simulink model "ramadan_2022"  (R2021a)
settings: Solver=ode15s  StartTime=0.0  StopTime=10  MaxStep=1e-2  MinStep=1e-20  RelTol=1e-3
StartFcn:
  | tic
StopFcn:
  | toc
  | 
  | 
  | %if GimbalLockFlag
  |  % fprintf(2, 'Almost reached Gimbal Lock of IMU. Simulation stopped.\n')
  | %end
  | 
  | %fprintf('Elapsed time: %4.2f sec (%4.2f%% realtime)\n', a, tout(end)/a*100)
values from neighbouring files (symbols this model uses):
  Balance = pMod(26:29)    [AssignSimulinkParams.m]    (also in assign_parameters.m = param(26:29))
  BalanceTrunkLat = pMod(22:25)    [AssignSimulinkParams.m]    (also in assign_parameters.m = param(22:25))
  BasisStim = pMod(1:11)    [AssignSimulinkParams.m]    (also in assign_parameters.m = param(1:11))
  CompliantLeg = pMod(12:14)    [AssignSimulinkParams.m]    (also in assign_parameters.m = param(12:14))
  CompliantLegLat = pMod(15)    [AssignSimulinkParams.m]    (also in assign_parameters.m = param(15))
  lp1 = 0.45    [nms3D_prep.m]
  lp2 = 0.55    [nms3D_prep.m]
  N = size(x,1)    [cmaes_hg.m]
  PreventKneeOverextension = pMod(16:21)    [AssignSimulinkParams.m]    (also in assign_parameters.m = param(16:21))
  propulsion = pMod(35)    [AssignSimulinkParams.m]    (also in assign_parameters.m = param(35))
  s = x(1:N-1,:).^2 + x(2:N,:).^2    [cmaes_hg.m]
  Target02 = pMod(30)    [AssignSimulinkParams.m]    (also in assign_parameters.m = param(30))
  Target13 = pMod(31:33)    [AssignSimulinkParams.m]    (also in assign_parameters.m = param(31:33))
  theta0 = pMod(34)    [AssignSimulinkParams.m]    (also in assign_parameters.m = param(34))
  WramameiSL_1000 = readmatrix('WSL_1000_Norm_Sigmoid_MSE_cont.csv')    [nms3D_prep.m]
  ZramameiSL_1000 = readmatrix('ZSL_1000_Norm_Sigmoid_MSE_cont.csv')    [nms3D_prep.m]
undefined symbols (not defined in the file or in its folder): ICs, mParams, X, Y, Z
libraries: nesl_utility x110, sm_lib x88, simulink x79, eeGeneralControl x28, robotmaniplib x10, dspinverses x10, robotcorelib x5, dspmathops x3, pid_lib x2, vrlib x1
(part 1 of 9)
settings Model: SimulationMode=rapid-accelerator  Creator=hgeyer  LastModifiedBy=rachidramadan
settings SolverCC: AlgebraicLoopSolver=TrustRegion  DecoupledContinuousIntegration=on  MinimalZcImpactIntegration=on
settings OptimizationCC: EfficientMapNaN2IntZero=off
settings DebuggingCC: ReadBeforeWriteMsg=DisableAll  WriteAfterWriteMsg=DisableAll  WriteAfterReadMsg=DisableAll  IgnoredZcDiagnostic=none  MultiTaskDSMMsg=none  SFMachineParentedDataDiag=warning  ArithmeticOperatorsInVariantConditions=warning
settings HardwareCC: TargetBitPerLong=64  TargetBitPerPointer=64  TargetBitPerSizeT=64  TargetBitPerPtrDiffT=64  TargetLongLongMode=on  TargetIntDivRoundTo=Zero  TargetEndianess=LittleEndian  TargetWordSize=64  TargetHWDeviceType=MATLAB Host  ProdEqTarget=off
settings ModelReferenceCC: UpdateModelReferenceTargets=IfOutOfDate
settings SFSimCC: SFSimEcho=off  SimUseLocalCustomCode=off  CustomCodeUndefinedFunction=UseInterfaceOnly
settings CodeAppCC: MaxIdLength=128
settings ConfigComp: CovScope=ReferencedModels
settings SimscapeCC: SimscapeNormalizeSystem=off
settings ExplorerConfigSet: InternalSimMechanicsExplorerSettings="<ExplorerConfiguration><canonicalview>planar_xy</canonicalview><AnimationSetting><BasePlaybackSpeed>1.0</BasePlaybackSpeed><PlaybackSpeedFactor>1.0</PlaybackSpeedFactor></AnimationSetting><TilePanel><TileInfo><Tiles Columns=\"1\" Count=\"1\" Rows=\"1\"><Column Weight=\"1\"/><Row Weight=\"1\"/><Tile Height=\"1\" Width=\"1\" X=\"0\" Y=\"0\"/></Tiles></TileInfo><SceneInfo><SceneViewer><BGColor><R>0.60000002384185791</R><G>0.60000002384185791</G><B>0.60000002384185791</B></BGColor><Camera><DoPerspective>off</DoPerspective><Position><X>0.597774143722594631</X><Y>0.919449529340500282</Y><Z>14.1815791267909113</Z></Position><Center><X>0.597774143722594631</X><Y>0.919449529340500282</Y><Z>3.38181724401920292e-07</Z></Center><Up><X>0</X><Y>1</Y><Z>0</Z></Up><ViewLimDist>1</ViewLimDist><YLim>1.30566284997374105</YLim><XLim>1.60885047805753101</XLim></Camera></SceneViewer></SceneInfo></TilePanel><MechEditorPanel><Cameras/><GfxPanelCameraMap/><VideoCreator><PlaybackSpeedRatio>1.0</PlaybackSpeedRatio><FrameRate>30</FrameRate><VideoFormat>Motion JPEG AVI</VideoFormat><FrameSize>auto</FrameSize></VideoCreator></MechEditorPanel></ExplorerConfiguration>"

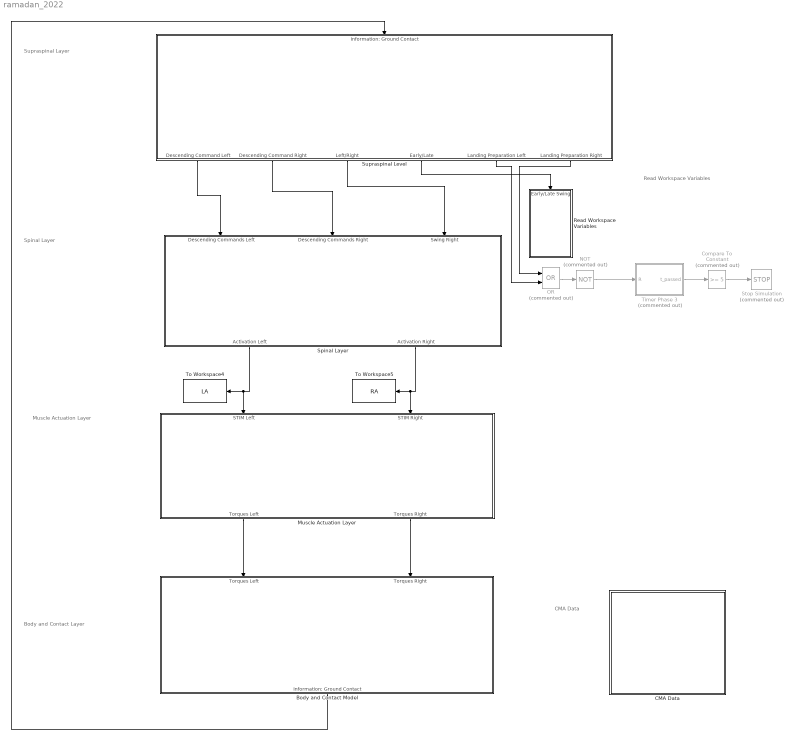
== system ramadan_2022 ==
  note: Spinal Layer
  note: Muscle Actuation Layer
  note: Body and Contact Layer
  note: Supraspinal Layer
  note: CMA Data
  note: Read Workspace Variables
  " Timer Phase 3" : Subsystem  Commented=on
  Body and Contact Model : Subsystem
  CMA Data : Subsystem
  Compare To Constant : simulink/Logic and Bit Operations/Compare To Constant  Commented=on  relop=>=  const=5  OutDataTypeStr=boolean  ZeroCross=off
  Muscle Actuation Layer : Subsystem
  NOT : Logic  Commented=on  Operator=NOT  AllPortsSameDT=off  OutDataTypeStr=boolean
  OR : Logic  Commented=on  Operator=OR  AllPortsSameDT=off  OutDataTypeStr=boolean
  Read Workspace Variables : Subsystem
  Spinal Layer : Subsystem
  Stop Simulation : Stop  Commented=on
  Supraspinal Level : Subsystem
  To Workspace4 : ToWorkspace  VariableName=LA  SampleTime=-1
      settings: Save2DSignal=2-D array (concatenate along first dimension)
  To Workspace5 : ToWorkspace  VariableName=RA  SampleTime=-1
      settings: Save2DSignal=2-D array (concatenate along first dimension)
  wires:
  Spinal Layer/1(Activation Left) -> To Workspace4/1, Muscle Actuation Layer/1(STIM Left)
  Spinal Layer/2(Activation Right) -> To Workspace5/1, Muscle Actuation Layer/2(STIM Right)
  Muscle Actuation Layer/2(Torques Right) -> Body and Contact Model/2(Torques Right)
  Supraspinal Level/1(Descending Command Left) -> Spinal Layer/1(Descending Commands Left)
  Supraspinal Level/2(Descending Command Right) -> Spinal Layer/2(Descending Commands Right)
  Body and Contact Model/1(Information: Ground Contact) -> Supraspinal Level/1(Information: Ground Contact)
  Supraspinal Level/3(Left/Right) -> Spinal Layer/3(Swing Right)
  Supraspinal Level/4(Early/Late) -> Read Workspace Variables/1(Early/Late Swing)
  Muscle Actuation Layer/1(Torques Left) -> Body and Contact Model/1(Torques Left)
  " Timer Phase 3"/1(t_passed) -> Compare To Constant/1
  Compare To Constant/1 -> Stop Simulation/1
  OR/1 -> NOT/1
  Supraspinal Level/6(Landing Preparation Right) -> OR/1
  Supraspinal Level/5(Landing Preparation Left) -> OR/2
  NOT/1 -> " Timer Phase 3"/1(R)

== system ramadan_2022/ Timer Phase 3 ==
  R : Inport
  Clock1 : Clock
  Clock3 : Clock
      settings: Decimation=4
  NOT : Logic  Operator=NOT  AllPortsSameDT=off  OutDataTypeStr=boolean
  Resettable Subsystem : Subsystem  TreatAsAtomicUnit=on
  Sum1 : Sum  Inputs=|+-  InputSameDT=on  SaturateOnIntegerOverflow=on  OutDataTypeStr=Inherit: Same as first input
  Switch2 : Switch  Criteria=u2 > Threshold  RndMeth=Zero
  t_passed : Outport  VectorParamsAs1DForOutWhenUnconnected=off
  wires:
  Clock1/1 -> Sum1/1
  Clock3/1 -> Switch2/3, Resettable Subsystem/1(In1)
  Sum1/1 -> t_passed/1
  R/1 -> NOT/1, Switch2/2
  Switch2/1 -> Sum1/2
  Resettable Subsystem/1(Out1) -> Switch2/1
  NOT/1 -> Resettable Subsystem/Enable

== system ramadan_2022/Body and Contact Model ==
  note: Rigid Body
  note: Contact Model
  note: Vestibular System
  Torques Left : Inport
  Torques Right : Inport  Port=2
  6-DOF Joint IC : sm_lib/Joints/6-DOF Joint  JointMode=Normal  SenseConstraintForce=off  SenseConstraintForceX=off  SenseConstraintForceY=off  SenseConstraintForceZ=off  SenseConstraintTorque=off  SenseConstraintTorqueX=off  SenseConstraintTorqueY=off  SenseConstraintTorqueZ=off  SenseTotalForce=off  SenseTotalForceX=off  SenseTotalForceY=off  SenseTotalForceZ=off  SenseTotalTorque=off  SenseTotalTorqueX=off  SenseTotalTorqueY=off  SenseTotalTorqueZ=off  CompositeWrenchDir=BaseOnFollower  CompositeWrenchFrame=FollowerFrame  PxEquilibriumPosition=0  PxEquilibriumPositionUnits=m  PxSpringStiffness=0  PxSpringStiffnessUnits=N/m  PxDampingCoefficient=0  PxDampingCoefficientUnits=N/(m/s)  PxTorqueActuationMode=NoTorque  PxMotionActuationMode=ComputedMotion  PxSensePosition=off  PxSenseVelocity=off  PxSenseAcceleration=off  PxSenseTorqueForce=off  PxSenseLowerLimitTorqueForce=off  PxSenseUpperLimitTorqueForce=off  PxLowerLimitSpecify=off  PxLowerLimitBound=-1  PxLowerLimitBoundUnits=m  PxLowerLimitStiffness=1e6  PxLowerLimitStiffnessUnits=N/m  PxLowerLimitDamping=1e3  PxLowerLimitDampingUnits=N/(m/s)  PxLowerLimitTransitionRegionWidth=1e-4  PxLowerLimitTransitionRegionWidthUnits=m  PxUpperLimitSpecify=off  PxUpperLimitBound=1  PxUpperLimitBoundUnits=m  PxUpperLimitStiffness=1e6  PxUpperLimitStiffnessUnits=N/m  PxUpperLimitDamping=1e3  PxUpperLimitDampingUnits=N/(m/s)  PxUpperLimitTransitionRegionWidth=1e-4  PxUpperLimitTransitionRegionWidthUnits=m  PxPositionTargetSpecify=on  PxPositionTargetPriority=High  PxPositionTargetValue=ICs.trunk.x0  PxPositionTargetValueUnits=m  PxVelocityTargetSpecify=on  PxVelocityTargetPriority=High  PxVelocityTargetValue=ICs.trunk.vx0  PxVelocityTargetValueUnits=m/s  PyEquilibriumPosition=0  PyEquilibriumPositionUnits=m  PySpringStiffness=0  PySpringStiffnessUnits=N/m  PyDampingCoefficient=0  PyDampingCoefficientUnits=N/(m/s)  PyTorqueActuationMode=NoTorque  PyMotionActuationMode=ComputedMotion  PySensePosition=off  PySenseVelocity=off  PySenseAcceleration=off  PySenseTorqueForce=off  PySenseLowerLimitTorqueForce=off  PySenseUpperLimitTorqueForce=off  PyLowerLimitSpecify=off  PyLowerLimitBound=-1  PyLowerLimitBoundUnits=m  PyLowerLimitStiffness=1e6  PyLowerLimitStiffnessUnits=N/m  PyLowerLimitDamping=1e3  PyLowerLimitDampingUnits=N/(m/s)  PyLowerLimitTransitionRegionWidth=1e-4  PyLowerLimitTransitionRegionWidthUnits=m  PyUpperLimitSpecify=off  PyUpperLimitBound=1  PyUpperLimitBoundUnits=m  PyUpperLimitStiffness=1e6  PyUpperLimitStiffnessUnits=N/m  PyUpperLimitDamping=1e3  PyUpperLimitDampingUnits=N/(m/s)  PyUpperLimitTransitionRegionWidth=1e-4  PyUpperLimitTransitionRegionWidthUnits=m  PyPositionTargetSpecify=on  PyPositionTargetPriority=High  PyPositionTargetValue=ICs.trunk.y0  PyPositionTargetValueUnits=m  PyVelocityTargetSpecify=off  PyVelocityTargetPriority=High  PyVelocityTargetValue=0  PyVelocityTargetValueUnits=m/s  PzEquilibriumPosition=0  PzEquilibriumPositionUnits=m  PzSpringStiffness=0  PzSpringStiffnessUnits=N/m  PzDampingCoefficient=0  PzDampingCoefficientUnits=N/(m/s)  PzTorqueActuationMode=NoTorque  PzMotionActuationMode=ComputedMotion  PzSensePosition=off  PzSenseVelocity=off  PzSenseAcceleration=off  PzSenseTorqueForce=off  PzSenseLowerLimitTorqueForce=off  PzSenseUpperLimitTorqueForce=off  PzLowerLimitSpecify=off  PzLowerLimitBound=-1  PzLowerLimitBoundUnits=m  PzLowerLimitStiffness=1e6  PzLowerLimitStiffnessUnits=N/m  PzLowerLimitDamping=1e3  PzLowerLimitDampingUnits=N/(m/s)  PzLowerLimitTransitionRegionWidth=1e-4  PzLowerLimitTransitionRegionWidthUnits=m  PzUpperLimitSpecify=off  PzUpperLimitBound=1  PzUpperLimitBoundUnits=m  PzUpperLimitStiffness=1e6  PzUpperLimitStiffnessUnits=N/m  PzUpperLimitDamping=1e3  PzUpperLimitDampingUnits=N/(m/s)  PzUpperLimitTransitionRegionWidth=1e-4  PzUpperLimitTransitionRegionWidthUnits=m  PzPositionTargetSpecify=on  PzPositionTargetPriority=High  PzPositionTargetValue=ICs.trunk.z0  PzPositionTargetValueUnits=m  PzVelocityTargetSpecify=on  PzVelocityTargetPriority=High  PzVelocityTargetValue=ICs.trunk.vz0  PzVelocityTargetValueUnits=m/s  SphDefPosRotationMethod=None  SphDefPosRotationAngleUnits=deg  SphDefPosRotationStandardAxis=+Z  SphDefPosRotationAngle=0.0  SphDefPosRotationArbitraryAxis=[0 0 1]  SphDefPosFollAlignAxisA=+X  SphDefPosBaseAlignAxisA=+Y  SphDefPosFollAlignAxisB=+Y  SphDefPosBaseAlignAxisB=+Z  SphDefPosRotationSequenceAxes=FollowerAxes  SphDefPosRotationSequence=XYX  SphDefPosRotationSequenceAngles=[0 0 0]  SphDefPosRotationSequenceAnglesUnits=deg  SphDefPosRotationMatrix=[1 0 0; 0 1 0; 0 0 1]  SphEqPosRotationMethod=None  SphEqPosRotationAngleUnits=deg  SphEqPosRotationStandardAxis=+Y  SphEqPosRotationAngle=0.0  SphEqPosRotationArbitraryAxis=[0 0 1]  SphEqPosFollAlignAxisA=+X  SphEqPosBaseAlignAxisA=+Y  SphEqPosFollAlignAxisB=+Y  SphEqPosBaseAlignAxisB=+Z  SphEqPosRotationSequenceAxes=FollowerAxes  SphEqPosRotationSequence=XYZ  SphEqPosRotationSequenceAngles=[0 0 -0.3]  SphEqPosRotationSequenceAnglesUnits=rad  SphEqPosRotationMatrix=[1 0 0; 0 1 0; 0 0 1]  SphSpringStiffness=0  SphSpringStiffnessUnits=N*m/deg  SphDampingCoefficient=0  SphDampingCoefficientUnits=N*m/(deg/s)  SphActuateTorqueX=off  SphActuateTorqueY=off  SphActuateTorqueZ=off  SphActuateTorque=on  SphTorqueActuationMode=NoTorque  SphMotionActuationMode=ComputedMotion  SphActuationFrame=BaseFrame  SphSensePosition=off  SphSenseVelocityX=off  SphSenseVelocityY=off  SphSenseVelocityZ=off  SphSenseVelocity=off  SphSenseAccelerationX=off  SphSenseAccelerationY=off  SphSenseAccelerationZ=off  SphSenseAcceleration=off  SphSenseTorqueX=off  SphSenseTorqueY=off  SphSenseTorqueZ=off  SphSenseTorqueForce=off  SphSenseLowerLimitTorqueMag=off  SphSenseUpperLimitTorqueMag=off  SphSensingFrame=BaseFrame  SphLowerLimitSpecify=off  SphLowerLimitBound=15  SphLowerLimitBoundUnits=deg  SphLowerLimitStiffness=1e4  SphLowerLimitStiffnessUnits=N*m/deg  SphLowerLimitDamping=10  SphLowerLimitDampingUnits=N*m/(deg/s)  SphLowerLimitTransitionRegionWidth=0.1  SphLowerLimitTransitionRegionWidthUnits=deg  SphUpperLimitSpecify=off  SphUpperLimitBound=45  SphUpperLimitBoundUnits=deg  SphUpperLimitStiffness=1e4  SphUpperLimitStiffnessUnits=N*m/deg  SphUpperLimitDamping=10  SphUpperLimitDampingUnits=N*m/(deg/s)  SphUpperLimitTransitionRegionWidth=0.1  SphUpperLimitTransitionRegionWidthUnits=deg  SphPositionTargetRotationMethod=RotationSequence  SphPositionTargetRotationAngleUnits=deg  SphPositionTargetRotationStandardAxis=+Z  SphPositionTargetRotationAngle=0.0  SphPositionTargetRotationArbitraryAxis=[0 0 1]  SphPositionTargetFollAlignAxisA=+X  SphPositionTargetBaseAlignAxisA=+Y  SphPositionTargetFollAlignAxisB=+Y  SphPositionTargetBaseAlignAxisB=+Z  SphPositionTargetRotationSequenceAxes=BaseAxes  SphPositionTargetRotationSequence=XZY  SphPositionTargetRotationSequenceAngles=[ICs.trunk.qR0 ICs.trunk.qP0 ICs.trunk.qY0 ]  SphPositionTargetRotationSequenceAnglesUnits=rad  SphPositionTargetRotationMatrix=[1 0 0; 0 1 0; 0 0 1]  SphPositionTargetSpecify=on  SphPositionTargetPriority=High  SphVelocityTargetValue=[ICs.trunk.qR0 ICs.trunk.qP0 ICs.trunk.qY0 ]  SphVelocityTargetValueUnits=deg/s  SphVelocityTargetSpecify=on  SphVelocityTargetPriority=High  SphVelocityTargetInFollowerFrame=on
  Clock : Clock
  Compare To Constant : simulink/Logic and Bit Operations/Compare To Constant  relop=<=  const=0.05  OutDataTypeStr=boolean
  Constant : Constant  Value=0
  External Force and Torque : sm_lib/Forces and Torques/External Force and Torque  ForceResolutionFrame=AttachedFrame  EnableForceX=on  EnableForceY=off  EnableForceZ=off  EnableForce=off  TorqueResolutionFrame=AttachedFrame  EnableTorqueX=off  EnableTorqueY=off  EnableTorqueZ=off  EnableTorque=off
  L Leg : Subsystem
  Minus : Sum  Inputs=-+
  PID Controller : pid_lib/PID Controller  Controller=P  Form=Parallel  TimeDomain=Continuous-time  UseExternalTs=off  SampleTime=-1  IntegratorMethod=Forward Euler  FilterMethod=Forward Euler  ControllerParametersSource=internal  P=7000  I=1  D=0  UseFilter=on  N=100  TunerSelectOption=Transfer Function Based (PID Tuner App)  ZeroCross=off  InitialConditionSource=internal  InitialConditionForIntegrator=0  InitialConditionForFilter=0  DifferentiatorICPrevScaledInput=0  ExternalReset=none  TrackingMode=off  Kt=1  LimitOutput=off  SatLimitsSource=internal  UpperSaturationLimit=inf  LowerSaturationLimit=-inf  LinearizeAsGain=on  AntiWindupMode=none  Kb=1  POutMin=[]  POutMax=[]  IOutMin=[]  IOutMax=[]  DOutMin=[]  DOutMax=[]  NOutMin=[]  NOutMax=[]  SumOutMin=[]  SumOutMax=[]  SaturationOutMin=[]  SaturationOutMax=[]  PParamMin=[]  PParamMax=[]  IParamMin=[]  IParamMax=[]  DParamMin=[]  DParamMax=[]  NParamMin=[]  NParamMax=[]  KbParamMin=[]  KbParamMax=[]  KtParamMin=[]  KtParamMax=[]  KbOutMin=[]  KbOutMax=[]  KtOutMin=[]  KtOutMax=[]  IntegratorOutMin=[]  IntegratorOutMax=[]  FilterOutMin=[]  FilterOutMax=[]  SumI1OutMin=[]  SumI1OutMax=[]  SumI2OutMin=[]  SumI2OutMax=[]  SumI3OutMin=[]  SumI3OutMax=[]  SumI4OutMin=[]  SumI4OutMax=[]  SumDOutMin=[]  SumDOutMax=[]  DifferentiatorOutMin=[]  DifferentiatorOutMax=[]  FilterDiffOutCoefMin=[]  FilterDiffOutCoefMax=[]  ReciprocalOutMin=[]  ReciprocalOutMax=[]  SumDenOutMin=[]  SumDenOutMax=[]  SumNumOutMin=[]  SumNumOutMax=[]  DivideOutMin=[]  DivideOutMax=[]  UdiffTsProdOutMin=[]  UdiffTsProdOutMax=[]  NTsProdOutMin=[]  NTsProdOutMax=[]  UintegralTsProdOutMin=[]  UintegralTsProdOutMax=[]  UngainTsProdOutMin=[]  UngainTsProdOutMax=[]  IntegratorContinuousStateAttributes=''  IntegratorStateMustResolveToSignalObject=off  IntegratorRTWStateStorageClass=Auto  FilterContinuousStateAttributes=''  FilterStateMustResolveToSignalObject=off  FilterRTWStateStorageClass=Auto  ParallelPVariant=InternalParameters  IdealPVariant=Disabled  IVariant=Disabled  DVariant=Disabled  IntegratorVariant=Disabled  SatVariant=Disabled  AWVariant=Disabled  PCopyVariant=Disabled  TRVariant=Disabled  FdbkBlocksVariant=Forward  IdealPFdbkVariant=Disabled  SatFdbkVariant=Disabled  DerivativeFilterVariant=Disabled  NVariant=Disabled  NCopyVariant=Disabled_SignalSpec  FilterICVariant=Disabled  IntegratorICVariant=Disabled  ExternalResetVariant=Disabled  TRSumVariant=Passthrough  SumFdbkVariant=Disabled  SumVariant=Passthrough_P  TsampFilterVariant=InternalTs  TsampNgainVariant=Passthrough  TsampIntegralVariant=Disabled_SignalSpec  ExternalSaturationOutDataTypeStr=Inherit: Same as second input
  R Leg : Subsystem
  Selector : Selector  InputPortWidth=3  IndexOptions=Index vector (dialog)  Indices=[1]  OutputSizes=1
  Sensor Left Ankle : Subsystem
  Sensor Left Ankle1 : Subsystem
  Simulink-PS Converter : nesl_utility/Simulink-PS Converter  PhysicalDomain=network_engine_domain  SubClassName=ps_input  LeftPortType=input  RightPortType=output  PseudoPeriodic=off  Frequencies=[]  NoiseDistribution=none  NoiseParameters=[]  Unit=1  AffineConversion=off  FilteringAndDerivatives=provide  SimscapeFilterOrder=1  InputFilterTimeConstant=0.001  UdotUserProvided=0
      settings: SourceProductBaseCode=PW,SS
  Subsystem : Subsystem
  Switch : Switch  Criteria=u2 > Threshold
  Terminator : Terminator
  Terminator1 : Terminator
  To Workspace1 : ToWorkspace  VariableName=Rlegq  SampleTime=-1
      settings: Save2DSignal=2-D array (concatenate along first dimension)
  To Workspace2 : ToWorkspace  VariableName=Llegdq  SampleTime=-1
      settings: Save2DSignal=2-D array (concatenate along first dimension)
  To Workspace3 : ToWorkspace  VariableName=Llegq  SampleTime=-1
      settings: Save2DSignal=2-D array (concatenate along first dimension)
  Trunk (floating base) : Subsystem
  Vestibular System : Subsystem
  World Frame : Subsystem
  Information: Ground Contact : Outport
  tag scope: LHL=global, LHR=global, Llegddq=global, Llegdq=global, Llegq=global, Rlegddq=global, Rlegdq=global, Rlegq=global
  wires:
  R Leg/4("Joint Velocities Right [rad/s] ") -> [Rlegdq]
  R Leg/5(Joint Accelerations Right [rad/s^2]) -> [Rlegddq]
  R Leg/3(Joint Angles Right [rad]) -> To Workspace1/1, [Rlegq]
  L Leg/3(Joint Angles Left [rad]) -> To Workspace3/1, [Llegq]
  L Leg/5(Joint Accelerations Left [rad/s^2]) -> [Llegddq]
  L Leg/4("Joint Velocities Left [rad/s] ") -> To Workspace2/1, [Llegdq]
  R Leg/2(Position Right Ankle [m]) -> Vestibular System/1(Ankle Position Right [m])
  L Leg/2(" Position Left Ankle [m]") -> Vestibular System/2(Ankle Position Left [m])
  Subsystem/1(Information: Ground Contact) -> Information: Ground Contact/1
  L Leg/1(Rotation Matrix Left Knee (world)) -> Terminator/1
  R Leg/1(Rotation Matrix Right Knee (World)) -> Terminator1/1
  Torques Right/1 -> R Leg/1(Torques [Nm])
  Torques Left/1 -> L Leg/1(Torques [Nm])
  Sensor Left Ankle/1(Position [m]) -> [LHL]
  Sensor Left Ankle1/1(Position [m]) -> [LHR]
  [CoM_Velocity] -> Selector/1
  Selector/1 -> Minus/1
  [v_init] -> Minus/2
  Minus/1 -> PID Controller/1
  PID Controller/1 -> Switch/1
  Constant/1 -> Switch/3
  Clock/1 -> Compare To Constant/1
  Compare To Constant/1 -> Switch/2
  Switch/1 -> Simulink-PS Converter/1
  connections:
  Trunk (floating base)/RConn1 -- Vestibular System/LConn3 -- L Leg/LConn1
  World Frame/RConn1 -- Subsystem/LConn1 -- 6-DOF Joint IC/LConn1
  L Leg/RConn1 -- Subsystem/RConn1
  L Leg/RConn2 -- Sensor Left Ankle/LConn1 -- Subsystem/RConn2
  L Leg/RConn3 -- Subsystem/RConn3
  L Leg/RConn4 -- Subsystem/RConn4
  R Leg/RConn3 -- Subsystem/RConn7
  R Leg/RConn4 -- Subsystem/RConn8
  Vestibular System/LConn2 -- R Leg/LConn1 -- Trunk (floating base)/RConn2
  6-DOF Joint IC/RConn1 -- Vestibular System/LConn1 -- Trunk (floating base)/LConn1 -- External Force and Torque/RConn1
  Subsystem/RConn6 -- Sensor Left Ankle1/LConn1 -- R Leg/RConn1
  R Leg/RConn2 -- Subsystem/RConn5
  External Force and Torque/LConn1 -- Simulink-PS Converter/RConn1

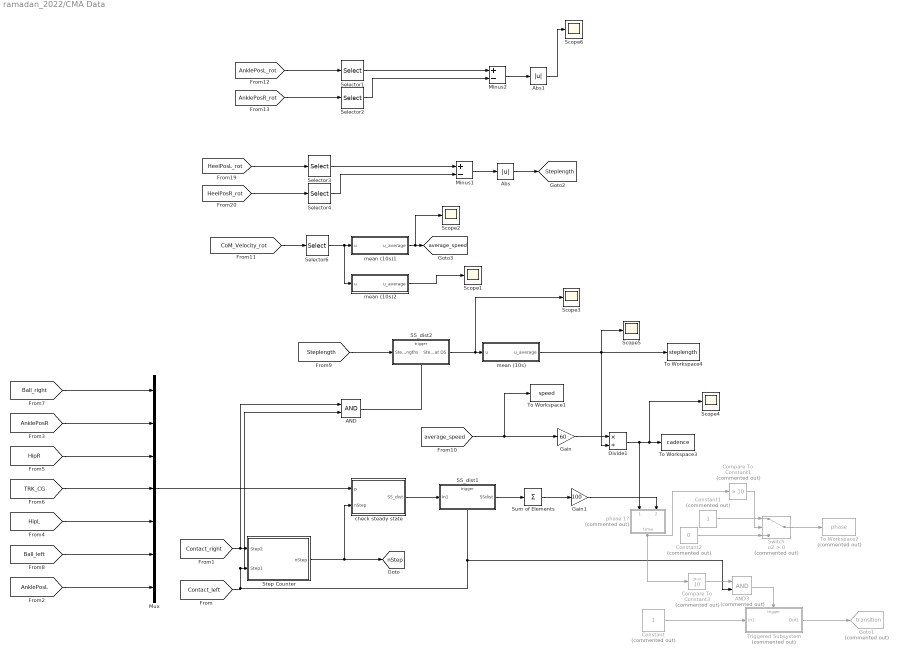
== system ramadan_2022/CMA Data ==
  AND : Logic  AllPortsSameDT=off  OutDataTypeStr=boolean
  AND3 : Logic  Commented=on  AllPortsSameDT=off  OutDataTypeStr=boolean
  Abs : Abs  ZeroCross=off
  Abs1 : Abs  ZeroCross=off
  Compare To Constant1 : simulink/Logic and Bit Operations/Compare To Constant  Commented=on  relop=>  const=10  OutDataTypeStr=boolean
  Compare To Constant3 : simulink/Logic and Bit Operations/Compare To Constant  Commented=on  relop=>=  const=10  OutDataTypeStr=boolean
  Constant : Constant  Commented=on  VectorParams1D=off  SampleTime=-1
  Constant1 : Constant  Commented=on
  Constant2 : Constant  Commented=on  Value=0
  Divide1 : Product  Inputs=*/
  Gain : Gain  Gain=60
  Gain1 : Gain  Gain=100
  Goto1 : Goto  Commented=on  GotoTag=transition  TagVisibility=global
  Minus1 : Sum  Inputs=+-
  Minus2 : Sum  Inputs=+-
  Mux : Mux  Inputs=7
  SS_dist1 : Subsystem  TreatAsAtomicUnit=on
  SS_dist2 : Subsystem  TreatAsAtomicUnit=on
  Scope{1..6} (6 alike) : Scope
  Selector{1..4,6} (5 alike) : Selector  InputPortWidth=3  IndexOptions=Index vector (dialog)  Indices=[1]  OutputSizes=1
  Step Counter : Subsystem
  Sum of Elements : Sum  Inputs=+
  Switch : Switch  Commented=on  Criteria=u2 > Threshold
  To Workspace1 : ToWorkspace  VariableName=speed  SampleTime=-1
      settings: Save2DSignal=2-D array (concatenate along first dimension)
  To Workspace2 : ToWorkspace  Commented=on  VariableName=phase  SampleTime=-1
      settings: Save2DSignal=2-D array (concatenate along first dimension)
  To Workspace3 : ToWorkspace  VariableName=cadence  SampleTime=-1
      settings: Save2DSignal=2-D array (concatenate along first dimension)
  To Workspace4 : ToWorkspace  VariableName=steplength  SampleTime=-1
      settings: Save2DSignal=2-D array (concatenate along first dimension)
  Triggered Subsystem : Subsystem  Commented=on  TreatAsAtomicUnit=on
  check steady state : Subsystem
  mean (10s) : Subsystem
  mean (10s)1 : Subsystem
  mean (10s)2 : Subsystem
  phase 1? : Subsystem  Commented=on
  tag scope: Steplength=global, average_speed=global, nStep=global
  wires:
  Step Counter/1(nStep) -> check steady state/2(nStep), [nStep]
  [Contact_left] -> AND/2, Step Counter/2(Step1), SS_dist1/Trigger, AND3/2
  [Contact_right] -> AND/1, Step Counter/1(Step2)
  [Ball_right] -> Mux/1
  [AnklePosR] -> Mux/2
  [HipR] -> Mux/3
  [TRK_CG] -> Mux/4
  [HipL] -> Mux/5
  [Ball_left] -> Mux/6
  [AnklePosL] -> Mux/7
  Mux/1 -> check steady state/1(p)
  check steady state/1(SS_dist) -> SS_dist1/1(In1)
  [Steplength] -> SS_dist2/1(Steplengths)
  SS_dist2/1(Steplength at DS) -> Scope3/1, mean (10s)/1(u)
  AND/1 -> SS_dist2/Trigger
  mean (10s)/1(u_average) -> Divide1/2, To Workspace4/1, Scope5/1
  [average_speed] -> To Workspace1/1, Gain/1
  Divide1/1 -> Scope4/1, To Workspace3/1, phase 1?/1(cadence)
  Gain/1 -> Divide1/1
  SS_dist1/1(SSdist) -> Sum of Elements/1
  Sum of Elements/1 -> Gain1/1
  Compare To Constant3/1 -> AND3/1
  AND3/1 -> Triggered Subsystem/Trigger
  Triggered Subsystem/1(Out1) -> Goto1/1
  Constant/1 -> Triggered Subsystem/1(In1)
  Gain1/1 -> phase 1?/2(stability)
  phase 1?/1(time) -> Compare To Constant1/1, Compare To Constant3/1
  Constant1/1 -> Switch/1
  Constant2/1 -> Switch/3
  Switch/1 -> To Workspace2/1
  Compare To Constant1/1 -> Switch/2
  Selector3/1 -> Minus1/1
  [HeelPosL_rot] -> Selector3/1
  Selector4/1 -> Minus1/2
  [HeelPosR_rot] -> Selector4/1
  Minus1/1 -> Abs/1
  Abs/1 -> [Steplength]
  [CoM_Velocity_rot] -> Selector6/1
  mean (10s)1/1(u_average) -> Scope2/1, [average_speed]
  Selector6/1 -> mean (10s)2/1(u), mean (10s)1/1(u)
  Selector2/1 -> Minus2/2
  Abs1/1 -> Scope6/1
  [AnklePosL_rot] -> Selector1/1
  [AnklePosR_rot] -> Selector2/1
  Selector1/1 -> Minus2/1
  Minus2/1 -> Abs1/1
  mean (10s)2/1(u_average) -> Scope1/1

== system ramadan_2022/Muscle Actuation Layer ==
  note: Muscle Actuation Layer
  STIM Left : Inport
  STIM Right : Inport  Port=2
  Muscles Left : Subsystem
  Muscles Right : Subsystem
  Mux : Mux
  Mux1 : Mux
  Torques Left : Outport
  Torques Right : Outport  Port=2
  tag scope: BalanceTorqueLeft=global, stance_torque_left_norm=global, stance_torque_right_norm=global
  wires:
  STIM Left/1 -> Muscles Left/1(STIM Left)
  STIM Right/1 -> Muscles Right/1(STIM Right)
  Muscles Left/1(tauHipPitchL) -> Mux/1
  Muscles Left/2(tauHipRollL) -> Mux/2
  Muscles Right/1(tauHipPitchR) -> Mux1/1
  Muscles Right/2(tauHipRollR) -> Mux1/2
  Muscles Left/4(tauHipAnkleL) -> Mux/4
  Muscles Right/3(tauKneeR) -> Mux1/3
  Muscles Left/3(tauKneeL) -> Mux/3
  Muscles Right/4(tauHipAnkleR) -> Mux1/4
  Mux/1 -> Torques Left/1
  Mux1/1 -> Torques Right/1
  Muscles Right/5(Leg Torque) -> [stance_torque_right_norm]
  Muscles Left/5("Leg Torque ") -> [stance_torque_left_norm]

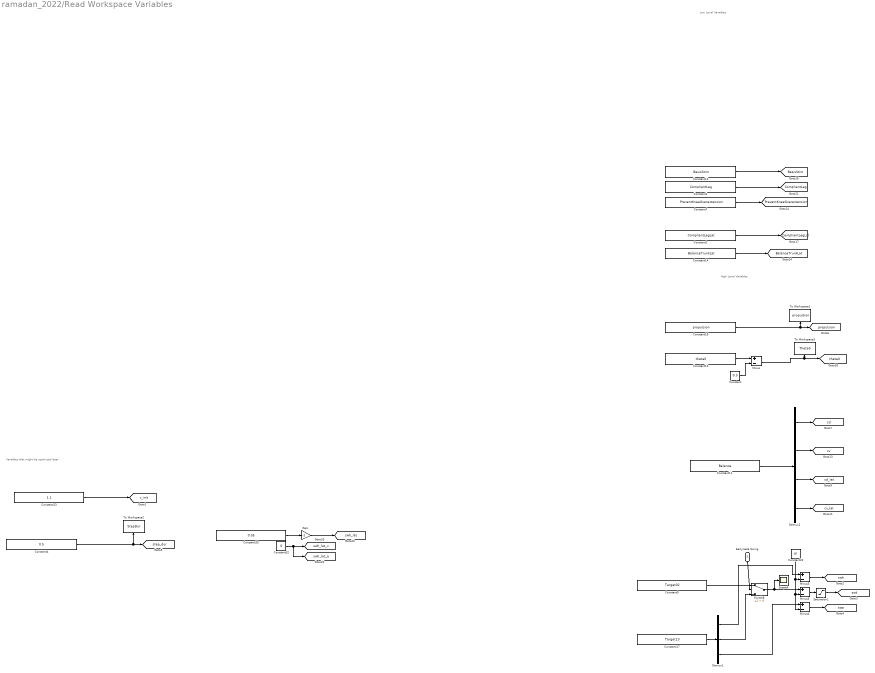
== system ramadan_2022/Read Workspace Variables ==
  note: Low Level Variables
  note: High Level Variables
  note: Variables that might be optimized later
  Early/Late Swing : Inport
  Constant : Constant  Value=0.3
  Constant1 : Constant  Value=CompliantLeg
  Constant10 : Constant  Value=theta0
  Constant11 : Constant  Value=Balance
  Constant12 : Constant  Value=BasisStim
  Constant14 : Constant  Value=BalanceTrunkLat
  Constant16 : Constant  Value=propulsion
  Constant17 : Constant  Value=Target13
  Constant2 : Constant  Value=CompliantLegLat
  Constant22 : Constant  Value=pi
  Constant23 : Constant  Value=1.1
  Constant32 : Constant  Value=0
  Constant33 : Constant  Value=0.05
  Constant4 : Constant  Value=0.5
  Constant7 : Constant  Value=PreventKneeOverextension
  Constant9 : Constant  Value=Target02
  Demux1 : Demux  Outputs=3
  Demux2 : Demux
  Gain : Gain  Gain=-1
  Minus{,3..5} (4 alike) : Sum  Inputs=+-
  Saturation1 : Saturate  UpperLimit=pi  LowerLimit=0  ZeroCross=off
  Scope4 : Scope
  Switch8 : Switch  Criteria=u2 > Threshold
  To Workspace1 : ToWorkspace  VariableName=propulsion  SampleTime=-1
      settings: Save2DSignal=2-D array (concatenate along first dimension)
  To Workspace2 : ToWorkspace  VariableName=StepDur  SampleTime=-1
      settings: Save2DSignal=2-D array (concatenate along first dimension)
  To Workspace3 : ToWorkspace  VariableName=Theta0  SampleTime=-1
      settings: Save2DSignal=2-D array (concatenate along first dimension)
  tag scope: BalanceTrunkLat=global, BasisStim=global, CompliantLeg=global, CompliantLegLat=global, PreventKneeOverextension=global, cd=global, cd_lat=global, cv=global, cv_lat=global, propulsion=global, step_dur=global, swa=global, swh=global, swh_lat=global, swh_lat_a=global, swh_lat_v=global, swk=global, theta0=global, v_init=global
  wires:
  Constant1/1 -> [CompliantLeg]
  Constant12/1 -> [BasisStim]
  Constant7/1 -> [PreventKneeOverextension]
  Demux2/3 -> [cd_lat]
  Demux2/2 -> [cv]
  Demux2/4 -> [cv_lat]
  Demux2/1 -> [cd]
  Constant2/1 -> [CompliantLegLat]
  Constant14/1 -> [BalanceTrunkLat]
  Constant33/1 -> Gain/1
  Constant16/1 -> [propulsion], To Workspace1/1
  Constant4/1 -> To Workspace2/1, [step_dur]
  Constant32/1 -> [swh_lat_a], [swh_lat_v]
  Gain/1 -> [swh_lat]
  Constant23/1 -> [v_init]
  Constant17/1 -> Demux1/1
  Constant9/1 -> Switch8/1
  Demux1/1 -> Minus3/1
  Demux1/2 -> Switch8/3
  Switch8/1 -> Minus5/1, Scope4/1
  Demux1/3 -> Minus4/1
  Minus3/1 -> [swh]
  Minus4/1 -> [swa]
  Constant22/1 -> Minus4/2, Minus5/2, Minus3/2
  Early/Late Swing/1 -> Switch8/2
  Constant11/1 -> Demux2/1
  Minus5/1 -> Saturation1/1
  Saturation1/1 -> [swk]
  Constant10/1 -> Minus/1
  Constant/1 -> Minus/2
  Minus/1 -> To Workspace3/1, [theta0]

== system ramadan_2022/Spinal Layer ==
  Descending Commands Left : Inport
  Descending Commands Right : Inport  Port=2
  Swing Right : Inport  Port=3
  Add1 : Sum
  Add2 : Sum
  Saturation1 : Saturate  UpperLimit=1  LowerLimit=0.001  ZeroCross=off
  Saturation2 : Saturate  UpperLimit=1  LowerLimit=0.001  ZeroCross=off
  Stance Leg Control Left : Subsystem
  Stance Leg Control Right : Subsystem
  Stretch Reflex for Swing Leg Control : Subsystem
  Switch : Switch  Criteria=u2 > Threshold
  Switch1 : Switch  Criteria=u2 > Threshold
  Activation Left : Outport
  Activation Right : Outport  Port=2
  wires:
  Descending Commands Right/1 -> Stretch Reflex for Swing Leg Control/2(Descending Commands Right)
  Descending Commands Left/1 -> Stretch Reflex for Swing Leg Control/1(Descending Commands Left)
  Stance Leg Control Left/1(Activation Left) -> Add1/2
  Stance Leg Control Right/1(Activation Right) -> Add2/2
  Switch1/1 -> Saturation1/1
  Switch/1 -> Saturation2/1
  Add1/1 -> Switch1/1
  Add2/1 -> Switch/3
  Saturation1/1 -> Activation Left/1
  Saturation2/1 -> Activation Right/1
  Stretch Reflex for Swing Leg Control/2(Activation Right) -> Add2/1, Switch/1
  Stretch Reflex for Swing Leg Control/1(Activation Left) -> Add1/1, Switch1/3
  Swing Right/1 -> Switch/2, Switch1/2, Stance Leg Control Right/1(Left/Right), Stance Leg Control Left/1(Left/Right)

== system ramadan_2022/Supraspinal Level ==
  note: Finite State Machine
  note: Computing Descending Commands for Swing Leg Control
  Information: Ground Contact : Inport
  Early/ Late : Logic  Operator=OR  AllPortsSameDT=off  OutDataTypeStr=boolean
  Finite State Machine : Subsystem
  Landing Preperation : Logic  Operator=OR  AllPortsSameDT=off  OutDataTypeStr=boolean
  Left/ Right : Logic  Operator=OR  Inputs=3  AllPortsSameDT=off  OutDataTypeStr=boolean
  Subsystem : Subsystem
  Terminator : Terminator
  To Workspace1 : ToWorkspace  VariableName=LateRight  SampleTime=-1
      settings: Save2DSignal=2-D array (concatenate along first dimension)
  To Workspace2 : ToWorkspace  VariableName=EarlyRight  SampleTime=-1
      settings: Save2DSignal=2-D array (concatenate along first dimension)
  To Workspace3 : ToWorkspace  VariableName=EarlyLeft  SampleTime=-1
      settings: Save2DSignal=2-D array (concatenate along first dimension)
  To Workspace4 : ToWorkspace  VariableName=Contact  SampleTime=-1
      settings: Save2DSignal=2-D array (concatenate along first dimension)
  Descending Command Left : Outport
  Descending Command Right : Outport  Port=2
  Left/Right : Outport  Port=3
  Early/Late : Outport  Port=4
  Landing Preparation Left : Outport  Port=5
  Landing Preparation Right : Outport  Port=6
  wires:
  Finite State Machine/3(Early Left Swing) -> Early/ Late/2, To Workspace3/1
  Finite State Machine/1(Early Right Swing) -> Left/ Right/1, Early/ Late/1, To Workspace2/1
  Finite State Machine/4(Late Left Swing) -> Terminator/1
  Finite State Machine/2(Late Right Swing) -> To Workspace1/1, Left/ Right/2
  Early/ Late/1 -> Subsystem/1(Early/Late Swing), Early/Late/1
  Information: Ground Contact/1 -> To Workspace4/1, Finite State Machine/1(Information: Ground Contact)
  Subsystem/1(Descending Command Left) -> Descending Command Left/1
  Subsystem/2(Descending Command Right) -> Descending Command Right/1
  Left/ Right/1 -> Left/Right/1, Subsystem/3(Swing Right)
  Finite State Machine/5(Landing Preparation Right) -> Landing Preperation/1, Left/ Right/3, Landing Preparation Right/1
  Finite State Machine/6(Landing Preparation Left) -> Landing Preparation Left/1, Landing Preperation/2
  Landing Preperation/1 -> Subsystem/2(Landing Preparation)

== system ramadan_2022/ Timer Phase 3/Resettable Subsystem ==
  In1 : Inport
  Enable : EnablePort  ZeroCross=off
  Out1 : Outport
  wires:
  In1/1 -> Out1/1
